simulink library "INT_SpdDemSwt_DD"  (R2016b)
settings: Solver=VariableStepAuto  StartTime=0.0  StopTime=10.0  RelTol=1e-3
settings Model: Creator=xuxingpei  LastModifiedBy=xuxingpei

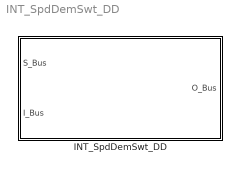
== system INT_SpdDemSwt_DD ==
  INT_SpdDemSwt_DD : Subsystem

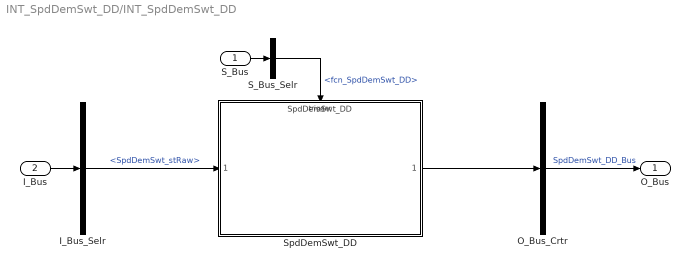
== system INT_SpdDemSwt_DD/INT_SpdDemSwt_DD ==
  S_Bus : Inport
  I_Bus : Inport  Port=2
  I_Bus_Selr : BusSelector  OutputSignals=SpdDemSwt_stRaw
  O_Bus_Crtr : BusCreator  Inputs=1
  S_Bus_Selr : BusSelector  OutputSignals=fcn_SpdDemSwt_DD
  SpdDemSwt_DD : ModelReference  ModelNameDialog=SpdDemSwt_DD  SimulationMode=Normal  ModelReferenceVersion=1.6  TriggerPortName=function  TriggerPortTriggerType=function-call  TriggerPortStatesWhenEnabling=held
  O_Bus : Outport
  wires:
  S_Bus_Selr/1 -> SpdDemSwt_DD/Trigger  "<fcn_SpdDemSwt_DD>"
  S_Bus/1 -> S_Bus_Selr/1
  I_Bus/1 -> I_Bus_Selr/1
  I_Bus_Selr/1 -> SpdDemSwt_DD/1  "<SpdDemSwt_stRaw>"
  O_Bus_Crtr/1 -> O_Bus/1  "SpdDemSwt_DD_Bus"
  SpdDemSwt_DD/1 -> O_Bus_Crtr/1
